simulink model "example_Hot_Water_Datafile"  (R2018b)
settings: Solver=ode45  StartTime=0.0  StopTime=7*24*3600  RelTol=1e-3  EnableMultiTasking=on
undefined symbols (not defined in the file): path_carnot
libraries: carnot x8
settings Model: Creator=drhf  LastModifiedBy=P41573
settings DataIOCC: LimitDataPoints=on  SaveFormat=Array  SignalLoggingSaveFormat=ModelDataLogs
settings OptimizationCC: ExpressionDepthLimit=2147483647  LifeSpan=inf
settings DebuggingCC: UnderspecifiedInitializationDetection=Classic  MergeDetectMultiDrivingBlocksExec=none  SolverPrmCheckMsg=warning  FcnCallInpInsideContextMsg=warning  StateNameClashWarn=warning  SFUnexpectedBacktrackingDiag=warning  SFNoUnconditionalDefaultTransitionDiag=warning  SFExecutionAtInitializationDiag=none
settings HardwareCC: ProdBitPerPointer=32  ProdBitPerSizeT=32  ProdBitPerPtrDiffT=32  ProdLargestAtomicFloat=None  ProdIntDivRoundTo=Undefined  ProdEndianess=Unspecified  ProdWordSize=32  ProdHWDeviceType=32-bit Generic
settings ModelReferenceCC: PropagateSignalLabelsOutOfModel=off
settings SFSimCC: SimUseLocalCustomCode=off
settings RTWCC: RTWUseLocalCustomCode=off
settings CodeAppCC: StateflowObjectComments=on
settings GRTTargetCC: TargetLangStandard=C89/C90 (ANSI)  GeneratePreprocessorConditionals=Disable all  CombineOutputUpdateFcns=off  GRTInterface=on
settings ConfigComp: CovMetricSettings=dw  CovHtmlReporting=on  CovSaveCumulativeToWorkspaceVar=on  CovSaveSingleToWorkspaceVar=on  CovExternalEMLEnable=off

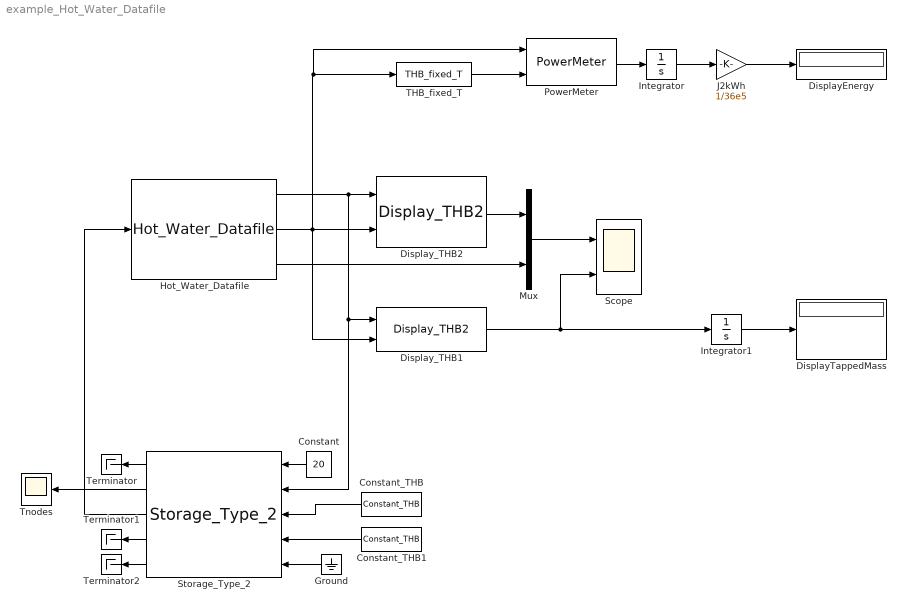
== system example_Hot_Water_Datafile ==
  Constant : Constant  Value=20
  Constant_THB : carnot/Source/Simple/Constant_THB  t=60  mdot=0.2  p=2e5  mID=No Pressure Drop  fluid=Water  mix=0  mix2=0  mix3=0  dia=0.02  hgt=0
      settings: SourceProductName=Carnot
  Constant_THB1 : carnot/Source/Simple/Constant_THB  t=60  mdot=0  p=2e5  mID=No Pressure Drop  fluid=Water  mix=0  mix2=0  mix3=0  dia=0.02  hgt=0
      settings: SourceProductName=Carnot
  DisplayEnergy : Display
  DisplayTappedMass : Display
  Display_THB1 : carnot/Outputs/Display_THB2  t=off  m=on  p=off  id=off  mix=off  d=off
      settings: SourceProductName=Carnot
  Display_THB2 : carnot/Outputs/Display_THB2  t=on  m=off  p=off  id=off  mix=off  d=off
      settings: SourceProductName=Carnot
  Ground : Ground
  Hot_Water_Datafile : carnot/Load/Hot_Water_Tapping/Hot_Water_Datafile  PathName=path_carnot('data')  FileName='DHWcalc_SFH_200L.mat'  Thot=45  Tcold=10  Tamp=3  dshift=-137
      settings: SourceProductName=Carnot
  Integrator : Integrator
  Integrator1 : Integrator
  J2kWh : Gain  Gain=1/36e5
  Mux : Mux  Inputs=2
  PowerMeter : carnot/Control/PowerMeter
      settings: SourceProductName=Carnot
  Scope : Scope  NumInputPorts=2
  Storage_Type_2 : carnot/Storage/Thermal/Storage_Type_2  t0=60  hgt=1.5279  stgtype=2  tini=[60 60 60 60 60 60 60 60 60 60]  mpts=[1 2 3 4 5 6 7 8 9 10]  PathName=fullfile(path_carnot('libsl'),'Storage','Thermal','Storage_Type_2','parameter_set')  FileName='StorageType2_300_L.mat'  userPath=off  userParam=off  uwall=1  ubot=1  utop=1  axcond=1  volume=0.3  dia=0.5  standing=standing cylinder  nodes=10  mpoints=10  Tsensor=0.5  hx1inlet=0.45  hx1outlet=0  hx1dia=0.03  hx1uac=50  hx1uam=0.15  hx1uat=0.6  uat2=0  hx1dpqua=20  hx1dplin=20  pipe1inlet=0  pipe1outlet=1  pipe1dia=0.03  pipe2inlet=0.6  pipe2outlet=1  pipe2dia=0.03  heater1start=0.6  heater1end=0.65
      settings: SourceProductName=Carnot
  THB_fixed_T : carnot/Source/Simple/THB_fixed_T  t=10
      settings: SourceProductName=Carnot
  Terminator : Terminator
  Terminator1 : Terminator
  Terminator2 : Terminator
  Tnodes : Scope
  wires:
  Display_THB2/1 -> Mux/1
  Hot_Water_Datafile/3 -> Mux/2
  Mux/1 -> Scope/1
  Display_THB1/1 -> Integrator1/1, Scope/2
  Storage_Type_2/3 -> Hot_Water_Datafile/1
  Hot_Water_Datafile/1 -> Storage_Type_2/2, Display_THB1/1, Display_THB2/1
  Storage_Type_2/1 -> Terminator/1
  Storage_Type_2/4 -> Terminator1/1
  Constant_THB/1 -> Storage_Type_2/3
  Constant/1 -> Storage_Type_2/1
  Storage_Type_2/2 -> Tnodes/1
  Hot_Water_Datafile/2 -> THB_fixed_T/1, PowerMeter/1, Display_THB1/2, Display_THB2/2
  PowerMeter/1 -> Integrator/1
  THB_fixed_T/1 -> PowerMeter/2
  Integrator/1 -> J2kWh/1
  J2kWh/1 -> DisplayEnergy/1
  Integrator1/1 -> DisplayTappedMass/1
  Storage_Type_2/5 -> Terminator2/1
  Constant_THB1/1 -> Storage_Type_2/4
  Ground/1 -> Storage_Type_2/5
